simulink model "fw_pos_control"  (R2024b)
settings: Solver=VariableStepAuto  StartTime=0.0  StopTime=10.0  RelTol=1e-3
undefined symbols (not defined in the file): FW_AIRSPD_MIN, FW_ARSP_MODE, FW_L1_DAMPING, FW_L1_PERIOD, FW_L1_R_SLEW_MAX, FW_POSCTL_INV_ST, FW_R_LIM, RWTO_AIRSPD_SCL, RWTO_RAMP_TIME
libraries: simulink_extras x10, matrix_library x7, simulink x3
settings Model: DataDictionary=nextpilot_datadict.sldd  Creator=CETCA  LastModifiedBy=cetca

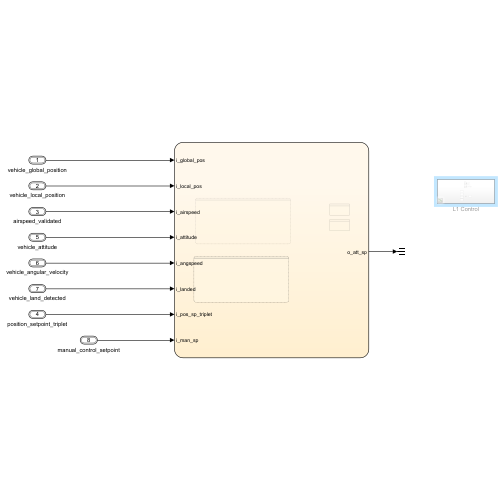
[thumbnail: Simulink's stored preview of the top-level diagram]
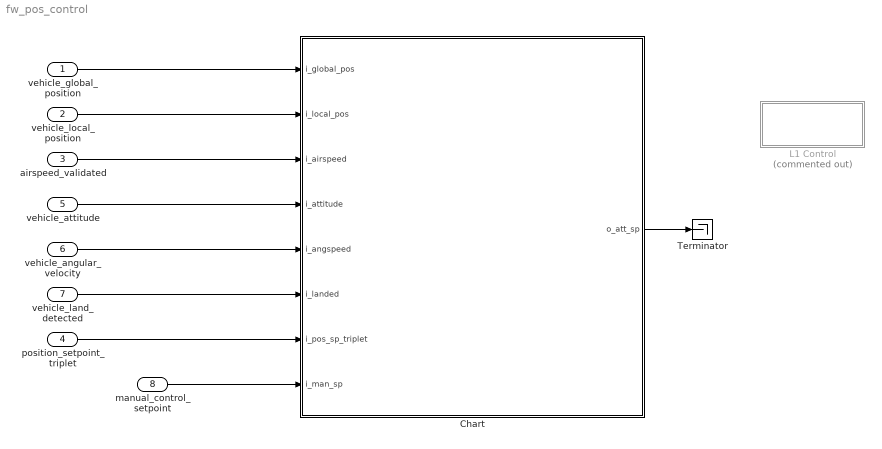
== system fw_pos_control ==
  vehicle_global_position : Inport  OutDataTypeStr=Bus: vehicle_global_position_s
  vehicle_local_position : Inport  Port=2  OutDataTypeStr=Bus: vehicle_local_position_s
  airspeed_validated : Inport  Port=3  OutDataTypeStr=Bus: airspeed_validated_s
  position_setpoint_triplet : Inport  Port=4  OutDataTypeStr=Bus: position_setpoint_triplet_s
  vehicle_attitude : Inport  Port=5  OutDataTypeStr=Bus: vehicle_attitude_s
  vehicle_angular_velocity : Inport  Port=6  OutDataTypeStr=Bus: vehicle_angular_velocity_s
  vehicle_land_detected : Inport  Port=7  OutDataTypeStr=Bus: vehicle_land_detected_s
  manual_control_setpoint : Inport  Port=8  OutDataTypeStr=Bus: manual_control_setpoint_s
  Chart : Stateflow chart  TreatAsAtomicUnit=on
  L1 Control : Subsystem  Commented=on
  Terminator : Terminator
  wires:
  vehicle_attitude/1 -> Chart/4(i_attitude)
  vehicle_angular_velocity/1 -> Chart/5(i_angspeed)
  vehicle_land_detected/1 -> Chart/6(i_landed)
  vehicle_global_position/1 -> Chart/1(i_global_pos)
  vehicle_local_position/1 -> Chart/2(i_local_pos)
  airspeed_validated/1 -> Chart/3(i_airspeed)
  position_setpoint_triplet/1 -> Chart/7(i_pos_sp_triplet)
  Chart/1(o_att_sp) -> Terminator/1
  manual_control_setpoint/1 -> Chart/8(i_man_sp)

== system fw_pos_control/Chart/L1.navigate_heading ==
  f : TriggerPort  TriggerType=function-call  VariantControl=(inherit)
      settings: CopyFcn=Stateflow.SLINSF.SimulinkMan.removeBlockPreDeleteFcn  PreDeleteFcn=Stateflow.SLINSF.SimulinkMan.unsafePredeleteFcn
  Ground : Ground
  nav_bearing : Outport
  bearing_error : Outport  Port=2
  target_bearing : Outport  Port=3
  wires:
  Ground/1 -> target_bearing/1, bearing_error/1, nav_bearing/1

== system fw_pos_control/Chart/L1.navigate_waypoints ==
  f : TriggerPort  TriggerType=function-call  VariantControl=(inherit)
      settings: CopyFcn=Stateflow.SLINSF.SimulinkMan.removeBlockPreDeleteFcn  PreDeleteFcn=Stateflow.SLINSF.SimulinkMan.unsafePredeleteFcn

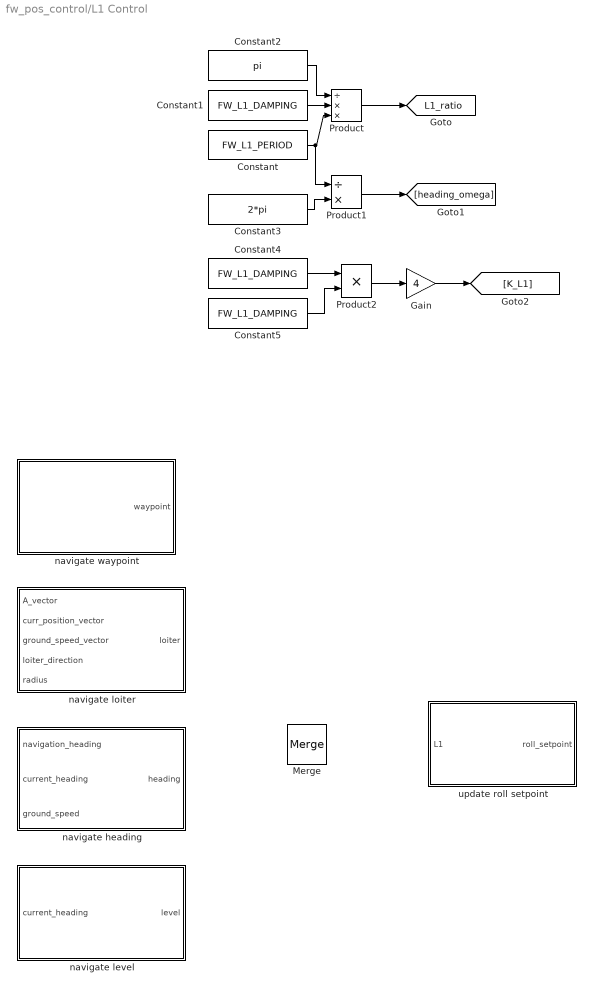
== system fw_pos_control/L1 Control ==
  Constant : Constant  Value=FW_L1_PERIOD
  Constant1 : Constant  Value=FW_L1_DAMPING
  Constant2 : Constant  Value=pi
  Constant3 : Constant  Value=2*pi
  Constant4 : Constant  Value=FW_L1_DAMPING
  Constant5 : Constant  Value=FW_L1_DAMPING
  Gain : Gain  Gain=4
  Merge : Merge  Inputs=4
  Product : Product  Inputs=/**
  Product1 : Product  Inputs=/*
  Product2 : Product
  navigate heading : Subsystem
  navigate level : Subsystem
  navigate loiter : Subsystem
  navigate waypoint : Subsystem
  update roll setpoint : Subsystem
  tag scope: L1_ratio=global
  wires:
  Constant2/1 -> Product/1
  Product/1 -> [L1_ratio]
  Constant1/1 -> Product/2
  Constant/1 -> Product1/1, Product/3
  Constant3/1 -> Product1/2
  Product1/1 -> [heading_omega]
  Constant4/1 -> Product2/1
  Constant5/1 -> Product2/2
  Product2/1 -> Gain/1
  Gain/1 -> [K_L1]

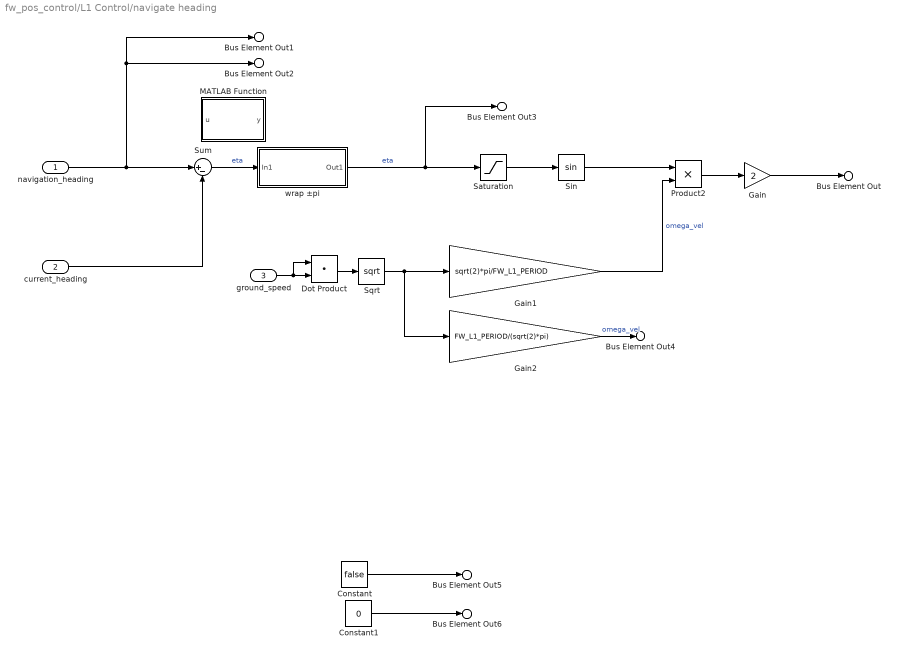
== system fw_pos_control/L1 Control/navigate heading ==
  navigation_heading : Inport
  current_heading : Inport  Port=2
  ground_speed : Inport  Port=3
  Constant : Constant  Value=false
  Constant1 : Constant  Value=0
  Dot Product : DotProduct  OutDataTypeStr=Inherit: Inherit via internal rule
  Gain : Gain  Gain=2
  Gain1 : Gain  Gain=sqrt(2)*pi/FW_L1_PERIOD
  Gain2 : Gain  Gain=FW_L1_PERIOD/(sqrt(2)*pi)
  MATLAB Function : MATLAB Function  TreatAsAtomicUnit=on
  Product2 : Product
  Saturation : Saturate  UpperLimit=pi/2  LowerLimit=-pi/2
      settings: AttributesFormatString=[%<LowerLimit>,%<UpperLimit>]
  Sin : Trigonometry
  Sqrt : Sqrt
  Sum : Sum  Inputs=|+-
  wrap ±pi : Subsystem
  Bus Element Out : Outport  PortName=heading  Element=lateral_accel
  Bus Element Out1 : Outport  PortName=heading  Element=target_bearing
  Bus Element Out2 : Outport  PortName=heading  Element=nav_bearing
  Bus Element Out3 : Outport  PortName=heading  Element=bearing_error
  Bus Element Out4 : Outport  PortName=heading  Element=L1_distance
  Bus Element Out5 : Outport  PortName=heading  Element=circle_mode
  Bus Element Out6 : Outport  PortName=heading  Element=crosstrack_error
  wires:
  navigation_heading/1 -> Bus Element Out2/1, Bus Element Out1/1, Sum/1
  current_heading/1 -> Sum/2
  wrap ±pi/1(Out1) -> Bus Element Out3/1, Saturation/1  "eta"
  Saturation/1 -> Sin/1
  ground_speed/1 -> Dot Product/2, Dot Product/1
  Sqrt/1 -> Gain2/1, Gain1/1
  Constant/1 -> Bus Element Out5/1
  Constant1/1 -> Bus Element Out6/1
  Sin/1 -> Product2/1
  Product2/1 -> Gain/1
  Sum/1 -> wrap ±pi/1(In1)  "eta"
  Dot Product/1 -> Sqrt/1
  Gain1/1 -> Product2/2  "omega_vel"
  Gain2/1 -> Bus Element Out4/1  "omega_vel"
  Gain/1 -> Bus Element Out/1

== system fw_pos_control/L1 Control/navigate level ==
  current_heading : Inport
  Constant : Constant  Value=false
  Constant1 : Constant  Value=0
  Bus Element Out : Outport  PortName=level  Element=target_bearing
  Bus Element Out1 : Outport  PortName=level  Element=nav_bearing
  Bus Element Out2 : Outport  PortName=level  Element=bearing_error
  Bus Element Out3 : Outport  PortName=level  Element=crosstrack_error
  Bus Element Out4 : Outport  PortName=level  Element=lateral_accel
  Bus Element Out5 : Outport  PortName=level  Element=circle_mode
  wires:
  Constant/1 -> Bus Element Out5/1
  Constant1/1 -> Bus Element Out3/1, Bus Element Out4/1, Bus Element Out2/1
  current_heading/1 -> Bus Element Out1/1, Bus Element Out/1

== system fw_pos_control/L1 Control/navigate loiter ==
  A_vector : Inport
  curr_position_vector : Inport  Port=2
  ground_speed_vector : Inport  Port=3
  loiter_direction : Inport  Port=4
  radius : Inport  Port=5
  Capture Mode : Subsystem
  Subsystem : Subsystem
  Bus Element Out : Outport  PortName=loiter  Element=signal1
  wires:
  ground_speed_vector/1 -> Subsystem/1(ground_speed_vector)
  Subsystem/1(guidance) -> Capture Mode/1(guidance)
  radius/1 -> Capture Mode/3(radius)
  loiter_direction/1 -> Capture Mode/2(loiter_direction)
  curr_position_vector/1 -> Subsystem/2(curr_position_vector)
  A_vector/1 -> Subsystem/3(coc_vector)

== system fw_pos_control/L1 Control/navigate waypoint ==
  Subsystem : Subsystem
  Subsystem1 : Subsystem
  Bus Element Out : Outport  PortName=waypoint  Element=signal1
  wires:
  Subsystem1/1(guidance) -> Subsystem/1(guidance)

== system fw_pos_control/L1 Control/update roll setpoint ==
  Bus Element In : Inport  PortName=L1  Element=lateral_accel
  Atan : Trigonometry  Operator=atan
  Gain : Gain  Gain=1/9.81
  Rate Limiter : RateLimiter  RisingSlewLimit=FW_L1_R_SLEW_MAX  FallingSlewLimit=-FW_L1_R_SLEW_MAX  SampleTimeMode=inherited
      settings: AttributesFormatString=[%<FallingSlewLimit>,%<RisingSlewLimit>]
  Saturation : Saturate  UpperLimit=FW_R_LIM  LowerLimit=-FW_R_LIM
      settings: AttributesFormatString=[%<LowerLimit>,%<UpperLimit>]
  roll_setpoint : Outport
  wires:
  Bus Element In/1 -> Gain/1
  Gain/1 -> Atan/1
  Atan/1 -> Saturation/1
  Saturation/1 -> Rate Limiter/1
  Rate Limiter/1 -> roll_setpoint/1

== system fw_pos_control/L1 Control/navigate heading/wrap ±pi ==
  In1 : Inport
  Bias : Bias  Bias=pi  SaturateOnIntegerOverflow=off
  Bias1 : Bias  Bias=-pi  SaturateOnIntegerOverflow=off
  Constant : Constant  Value=2*pi
  Mod : Math  Operator=mod
  Out1 : Outport
  wires:
  In1/1 -> Bias/1
  Bias/1 -> Mod/1
  Constant/1 -> Mod/2
  Mod/1 -> Bias1/1
  Bias1/1 -> Out1/1

== system fw_pos_control/L1 Control/navigate loiter/Capture Mode ==
  Bus Element In : Inport  PortName=guidance
  Bus Element In1 : Inport  PortName=guidance
  loiter_direction : Inport  Port=2
  radius : Inport  Port=3
  Check Switch Over : Subsystem
  Switch : Switch  Criteria=u2 > Threshold  SaturateOnIntegerOverflow=off  InputSameDT=off
  capture (towards waypoint center) : Subsystem
  circle (loiter) : Subsystem
  loiter_direction1 : InportShadow  Port=2
  Out1 : Outport
  wires:
  Check Switch Over/1(checkover) -> Switch/2
  capture (towards waypoint center)/1(capture) -> Check Switch Over/1(capture), Switch/1
  circle (loiter)/1(loiter) -> Check Switch Over/3(loiter), Switch/3
  Bus Element In/1 -> capture (towards waypoint center)/1(guidance)
  Bus Element In1/1 -> circle (loiter)/1(guidance)
  loiter_direction/1 -> Check Switch Over/2(direction)
  loiter_direction1/1 -> circle (loiter)/3(loiter_direction)
  radius/1 -> circle (loiter)/2(radius)
  Switch/1 -> Out1/1

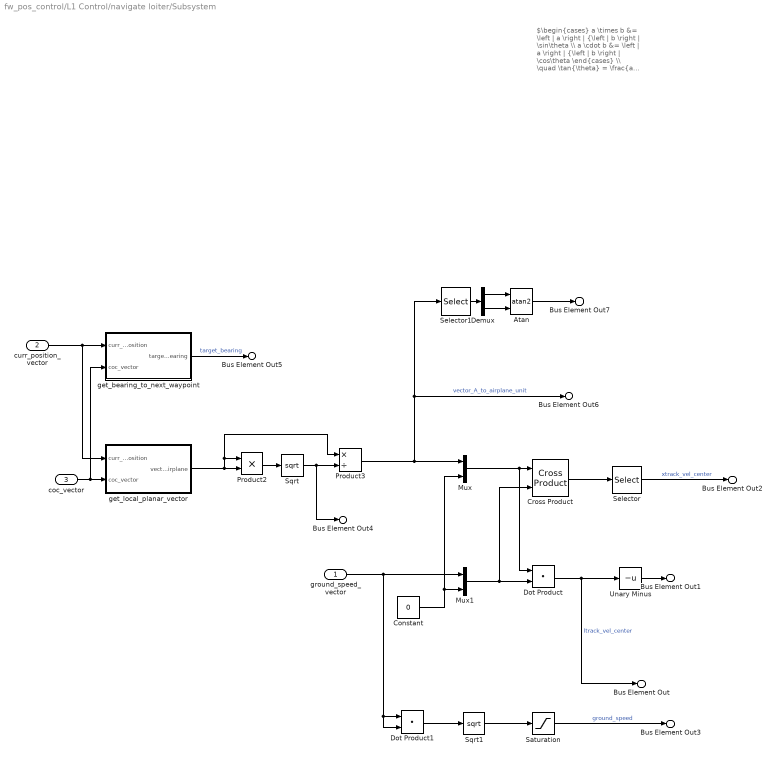
== system fw_pos_control/L1 Control/navigate loiter/Subsystem ==
  note: $\begin{cases} a \times b &= \left | a \right | {\left | b \right | \sin\theta \\ a \cdot b &= \left | a \right | {\left | b \right | \cos\theta \end{cases} \\ \quad \tan{\theta} = \frac{a \times b}{a \cdot b}$
  ground_speed_vector : Inport
  curr_position_vector : Inport  Port=2
  coc_vector : Inport  Port=3
  Atan : Trigonometry  Operator=atan2
  Constant : Constant  Value=0  OutDataTypeStr=single
  Cross Product : matrix_library/Cross Product
  Demux : Demux  Outputs=2
  Dot Product : DotProduct  OutDataTypeStr=Inherit: Inherit via internal rule
  Dot Product1 : DotProduct  OutDataTypeStr=Inherit: Inherit via internal rule
  Mux : Mux  Inputs=2
  Mux1 : Mux  Inputs=2
  Product2 : Product
  Product3 : Product  Inputs=*/
  Saturation : Saturate  UpperLimit=inf  LowerLimit=0.1
  Selector : Selector  InputPortWidth=3  IndexOptions=Index vector (dialog)  Indices=3  OutputSizes=1
  Selector1 : Selector  InputPortWidth=2  IndexOptions=Index vector (dialog)  Indices=[2 1]  OutputSizes=1
  Sqrt : Sqrt
  Sqrt1 : Sqrt
  Unary Minus : UnaryMinus
  get_bearing_to_next_waypoint : Subsystem
  get_local_planar_vector : Subsystem
  Bus Element Out : Outport  PortName=guidance  Element=xtrack_vel_circle
  Bus Element Out1 : Outport  PortName=guidance  Element=ltrack_vel_center
  Bus Element Out2 : Outport  PortName=guidance  Element=xtrack_vel_center
  Bus Element Out3 : Outport  PortName=guidance  Element=ground_speed
  Bus Element Out4 : Outport  PortName=guidance  Element=vector_A_to_airplane_length
  Bus Element Out5 : Outport  PortName=guidance  Element=target_bearing
  Bus Element Out6 : Outport  PortName=guidance  Element=vector_A_to_airplane_unit
  Bus Element Out7 : Outport  PortName=guidance  Element=nav_bearing
  wires:
  Dot Product/1 -> Bus Element Out/1, Unary Minus/1  "ltrack_vel_center"
  Unary Minus/1 -> Bus Element Out1/1
  Selector/1 -> Bus Element Out2/1  "xtrack_vel_center"
  Product3/1 -> Selector1/1, Bus Element Out6/1, Mux/1  "vector_A_to_airplane_unit"
  ground_speed_vector/1 -> Dot Product1/2, Dot Product1/1, Mux1/1
  Constant/1 -> Mux/2, Mux1/2
  Mux/1 -> Dot Product/1, Cross Product/1
  Mux1/1 -> Cross Product/2, Dot Product/2
  Cross Product/1 -> Selector/1
  get_local_planar_vector/1(vector_A_to_airplane) -> Product3/1, Product2/1, Product2/2
  Sqrt/1 -> Bus Element Out4/1, Product3/2
  Product2/1 -> Sqrt/1
  Dot Product1/1 -> Sqrt1/1
  Sqrt1/1 -> Saturation/1
  Saturation/1 -> Bus Element Out3/1  "ground_speed"
  get_bearing_to_next_waypoint/1(target_bearing) -> Bus Element Out5/1  "target_bearing"
  curr_position_vector/1 -> get_local_planar_vector/1(curr_position), get_bearing_to_next_waypoint/1(curr_position)
  coc_vector/1 -> get_bearing_to_next_waypoint/2(coc_vector), get_local_planar_vector/2(coc_vector)
  Selector1/1 -> Demux/1
  Demux/1 -> Atan/1
  Demux/2 -> Atan/2
  Atan/1 -> Bus Element Out7/1

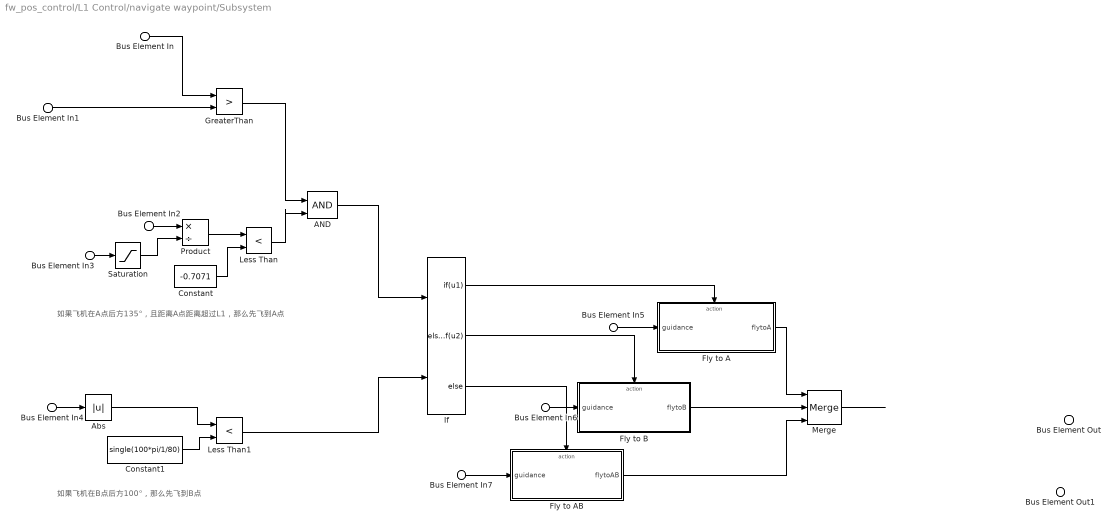
== system fw_pos_control/L1 Control/navigate waypoint/Subsystem ==
  note: 如果飞机在A点后方135°，且距离A点距离超过L1，那么先飞到A点
  note: 如果飞机在B点后方100°，那么先飞到B点
  Bus Element In5 : Inport  PortName=guidance
  Bus Element In6 : Inport  PortName=guidance
  Bus Element In7 : Inport  PortName=guidance
  Bus Element In : Inport  PortName=guidance  Element=distance_A_to_airplane
  Bus Element In3 : Inport  PortName=guidance  Element=distance_A_to_airplane
  Bus Element In2 : Inport  PortName=guidance  Element=alongTrackDist
  Bus Element In4 : Inport  PortName=guidance  Element=AB_to_BP_bearing
  Bus Element In1 : Inport  PortName=guidance  Element=L1_distance
  AND : Logic  IconShape=distinctive  AllPortsSameDT=off  OutDataTypeStr=boolean
  Abs : Abs  SaturateOnIntegerOverflow=off
  Constant : Constant  Value=-0.7071  OutDataTypeStr=single
  Constant1 : Constant  Value=single(100*pi/1/80)  OutDataTypeStr=single
  Fly to A : Subsystem  TreatAsAtomicUnit=on
  Fly to AB : Subsystem  TreatAsAtomicUnit=on
  Fly to B : Subsystem  TreatAsAtomicUnit=on
  GreaterThan : RelationalOperator  Operator=>  OutDataTypeStr=boolean  RndMeth=Simplest  InputSameDT=off
  If : If  NumInputs=2  IfExpression=u1  ElseIfExpressions=u2
  Less Than : RelationalOperator  Operator=<  OutDataTypeStr=boolean  RndMeth=Simplest  InputSameDT=off
  Less Than1 : RelationalOperator  Operator=<  OutDataTypeStr=boolean  RndMeth=Simplest  InputSameDT=off
  Merge : Merge  Inputs=3
  Product : Product  Inputs=*/
  Saturation : Saturate  UpperLimit=inf  LowerLimit=1
  Bus Element Out : Outport  PortName=OutBus  Element=bearing_error
  Bus Element Out1 : Outport  PortName=OutBus  Element=bearing_error1
  wires:
  Bus Element In/1 -> GreaterThan/1
  Bus Element In2/1 -> Product/1
  Bus Element In3/1 -> Saturation/1
  Saturation/1 -> Product/2
  Product/1 -> Less Than/1
  Constant/1 -> Less Than/2
  GreaterThan/1 -> AND/1
  Less Than/1 -> AND/2
  Bus Element In4/1 -> Abs/1
  Constant1/1 -> Less Than1/2
  Less Than1/1 -> If/2
  AND/1 -> If/1
  If/1 -> Fly to A/Action
  If/2 -> Fly to B/Action
  If/3 -> Fly to AB/Action
  Abs/1 -> Less Than1/1
  Bus Element In5/1 -> Fly to A/1(guidance)
  Bus Element In6/1 -> Fly to B/1(guidance)
  Bus Element In7/1 -> Fly to AB/1(guidance)
  Fly to A/1(flytoA) -> Merge/1
  Fly to B/1(flytoB) -> Merge/2
  Fly to AB/1(flytoAB) -> Merge/3
  Bus Element In1/1 -> GreaterThan/2
  Merge/1 -> ?

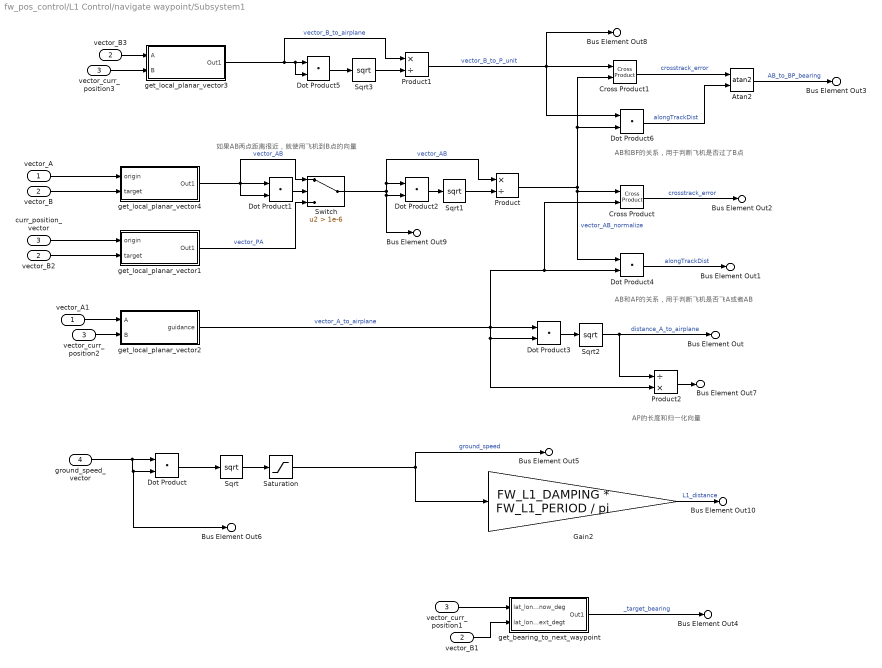
== system fw_pos_control/L1 Control/navigate waypoint/Subsystem1 ==
  note: AP的长度和归一化向量
  note: AB和AP的关系，用于判断飞机是否飞A或者AB
  note: AB和BP的关系，用于判断飞机是否过了B点
  note: 如果AB两点距离很近，就使用飞机到B点的向量
  vector_A : Inport
  vector_B : Inport  Port=2
  curr_position_vector : Inport  Port=3
  ground_speed_vector : Inport  Port=4
  Atan2 : Trigonometry  Operator=atan2
  Cross Product : matrix_library/Cross Product
  Cross Product1 : matrix_library/Cross Product
  Dot Product{,1..6} (7 alike) : DotProduct  OutDataTypeStr=Inherit: Inherit via internal rule
  Gain2 : Gain  Gain=FW_L1_DAMPING * FW_L1_PERIOD / pi
  Product : Product  Inputs=*/
  Product1 : Product  Inputs=*/
  Product2 : Product  Inputs=/*
  Saturation : Saturate  UpperLimit=inf  LowerLimit=0.1
  Sqrt{,1..3} (4 alike) : Sqrt
  Switch : Switch  Criteria=u2 > Threshold  Threshold=1e-6  SaturateOnIntegerOverflow=off  InputSameDT=off
  get_bearing_to_next_waypoint : Subsystem
  get_local_planar_vector1 : Subsystem
  get_local_planar_vector2 : Subsystem
  get_local_planar_vector3 : Subsystem
  get_local_planar_vector4 : Subsystem
  vector_A1 : InportShadow
  vector_B1 : InportShadow  Port=2
  vector_B2 : InportShadow  Port=2
  vector_B3 : InportShadow  Port=2
  vector_curr_position1 : InportShadow  Port=3
  vector_curr_position2 : InportShadow  Port=3
  vector_curr_position3 : InportShadow  Port=3
  Bus Element Out : Outport  PortName=guidance  Element=distance_A_to_airplane
  Bus Element Out1 : Outport  PortName=guidance  Element=alongTrackDist
  Bus Element Out2 : Outport  PortName=guidance  Element=crosstrack_error
  Bus Element Out3 : Outport  PortName=guidance  Element=AB_to_BP_bearing
  Bus Element Out5 : Outport  PortName=guidance  Element=ground_speed
  Bus Element Out6 : Outport  PortName=guidance  Element=ground_speed_vector
  Bus Element Out7 : Outport  PortName=guidance  Element=vector_A_to_airplane_unit
  Bus Element Out8 : Outport  PortName=guidance  Element=vector_B_to_P_unit
  Bus Element Out9 : Outport  PortName=guidance  Element=vector_AB
  Bus Element Out4 : Outport  PortName=guidance  Element=target_bearing
  Bus Element Out10 : Outport  PortName=guidance  Element=L1_distance
  wires:
  ground_speed_vector/1 -> Bus Element Out6/1, Dot Product/2, Dot Product/1
  Dot Product/1 -> Sqrt/1
  Sqrt/1 -> Saturation/1
  Saturation/1 -> Gain2/1, Bus Element Out5/1  "ground_speed"
  vector_B/1 -> get_local_planar_vector4/2(target)
  get_local_planar_vector4/1(Out1) -> Dot Product1/2, Switch/1, Dot Product1/1  "vector_AB"
  vector_curr_position1/1 -> get_bearing_to_next_waypoint/1(lat_lon_now_deg)
  vector_B1/1 -> get_bearing_to_next_waypoint/2(lat_lon_next_degt)
  get_bearing_to_next_waypoint/1(Out1) -> Bus Element Out4/1  "_target_bearing"
  vector_A/1 -> get_local_planar_vector4/1(origin)
  curr_position_vector/1 -> get_local_planar_vector1/1(origin)
  vector_B2/1 -> get_local_planar_vector1/2(target)
  get_local_planar_vector1/1(Out1) -> Switch/3  "vector_PA"
  Dot Product1/1 -> Switch/2
  Switch/1 -> Dot Product2/1, Product/1, Bus Element Out9/1, Dot Product2/2  "vector_AB"
  Dot Product2/1 -> Sqrt1/1
  Sqrt1/1 -> Product/2
  Product/1 -> Dot Product4/1, Cross Product/1, Dot Product6/2, Cross Product1/2  "vector_AB_normalize"
  vector_A1/1 -> get_local_planar_vector2/1(A)
  vector_curr_position2/1 -> get_local_planar_vector2/2(B)
  get_local_planar_vector2/1(guidance) -> Product2/2, Dot Product3/2, Cross Product/2, Dot Product4/2, Dot Product3/1  "vector_A_to_airplane"
  Cross Product/1 -> Bus Element Out2/1  "crosstrack_error"
  Dot Product3/1 -> Sqrt2/1
  Sqrt2/1 -> Product2/1, Bus Element Out/1  "distance_A_to_airplane"
  Dot Product4/1 -> Bus Element Out1/1  "alongTrackDist"
  vector_B3/1 -> get_local_planar_vector3/1(A)
  vector_curr_position3/1 -> get_local_planar_vector3/2(B)
  get_local_planar_vector3/1(Out1) -> Product1/1, Dot Product5/2, Dot Product5/1  "vector_B_to_airplane"
  Dot Product5/1 -> Sqrt3/1
  Sqrt3/1 -> Product1/2
  Product1/1 -> Bus Element Out8/1, Cross Product1/1, Dot Product6/1  "vector_B_to_P_unit"
  Cross Product1/1 -> Atan2/1  "crosstrack_error"
  Dot Product6/1 -> Atan2/2  "alongTrackDist"
  Atan2/1 -> Bus Element Out3/1  "AB_to_BP_bearing"
  Product2/1 -> Bus Element Out7/1
  Gain2/1 -> Bus Element Out10/1  "L1_distance"

== system fw_pos_control/L1 Control/navigate loiter/Capture Mode/Check Switch Over ==
  Bus Element In : Inport  PortName=capture  Element=lateral_accel
  direction : Inport  Port=2
  Bus Element In1 : Inport  Port=3  PortName=loiter  Element=lateral_accel
  Bus Element In2 : Inport  Port=3  PortName=loiter  Element=xtrack_err_circle
  AND : Logic  IconShape=distinctive  AllPortsSameDT=off  OutDataTypeStr=boolean
  Compare To Zero : simulink/Logic and Bit Operations/Compare To Zero  relop=>  OutDataTypeStr=boolean
  Compare To Zero1 : simulink/Logic and Bit Operations/Compare To Zero  relop=>  OutDataTypeStr=boolean
  Product8 : Product
  Sum : Sum  Inputs=|+-
  checkover : Outport
  wires:
  Product8/1 -> Compare To Zero/1
  Compare To Zero/1 -> AND/1
  direction/1 -> Product8/2
  Compare To Zero1/1 -> AND/2
  AND/1 -> checkover/1
  Bus Element In1/1 -> Sum/1
  Bus Element In/1 -> Sum/2
  Sum/1 -> Product8/1
  Bus Element In2/1 -> Compare To Zero1/1

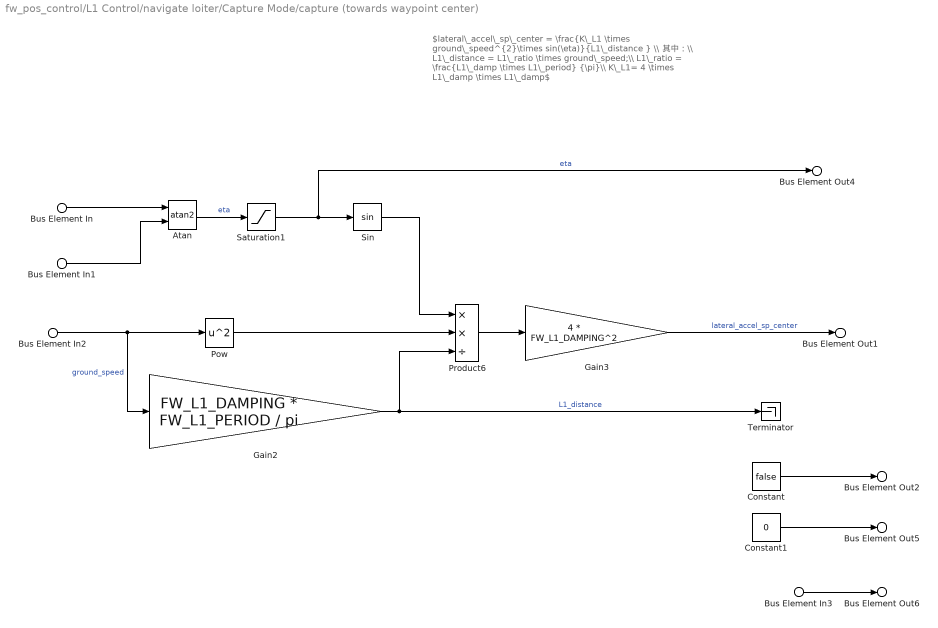
== system fw_pos_control/L1 Control/navigate loiter/Capture Mode/capture (towards waypoint center) ==
  note: $lateral\_accel\_sp\_center = \frac{K\_L1 \times ground\_speed^{2}\times sin(\eta)}{L1\_distance } \\ 其中：\\ L1\_distance = L1\_ratio \times ground\_speed;\\ L1\_ratio = \frac{L1\_damp \times L1\_period} {\pi}\\ K\_L1= 4 \times L1\_damp \times L1\_damp$
  Bus Element In : Inport  PortName=guidance  Element=xtrack_vel_center
  Bus Element In1 : Inport  PortName=guidance  Element=ltrack_vel_center
  Bus Element In2 : Inport  PortName=guidance  Element=ground_speed
  Bus Element In3 : Inport  PortName=guidance  Element=nav_bearing
  Atan : Trigonometry  Operator=atan2
  Constant : Constant  Value=false
  Constant1 : Constant  Value=0
  Gain2 : Gain  Gain=FW_L1_DAMPING * FW_L1_PERIOD / pi
  Gain3 : Gain  Gain=4 * FW_L1_DAMPING^2
  Pow : Math  Operator=square  SignedPower=on  RndMeth=Zero
  Product6 : Product  Inputs=**/
  Saturation1 : Saturate  UpperLimit=single(pi/2)  LowerLimit=-single(pi/2)
      settings: AttributesFormatString=[%<LowerLimit>,%<UpperLimit>]
  Sin : Trigonometry
  Terminator : Terminator
  Bus Element Out2 : Outport  PortName=capture  Element=circle_mode
  Bus Element Out1 : Outport  PortName=capture  Element=lateral_accel
  Bus Element Out4 : Outport  PortName=capture  Element=bearing_error
  Bus Element Out6 : Outport  PortName=capture  Element=nav_bearing
  Bus Element Out5 : Outport  PortName=capture  Element=xtrack_err_circle
  wires:
  Sin/1 -> Product6/1
  Saturation1/1 -> Bus Element Out4/1, Sin/1  "eta"
  Bus Element In2/1 -> Pow/1, Gain2/1  "ground_speed"
  Gain2/1 -> Terminator/1, Product6/3  "L1_distance"
  Gain3/1 -> Bus Element Out1/1  "lateral_accel_sp_center"
  Bus Element In1/1 -> Atan/2
  Pow/1 -> Product6/2
  Atan/1 -> Saturation1/1  "eta"
  Product6/1 -> Gain3/1
  Bus Element In/1 -> Atan/1
  Constant/1 -> Bus Element Out2/1
  Constant1/1 -> Bus Element Out5/1
  Bus Element In3/1 -> Bus Element Out6/1

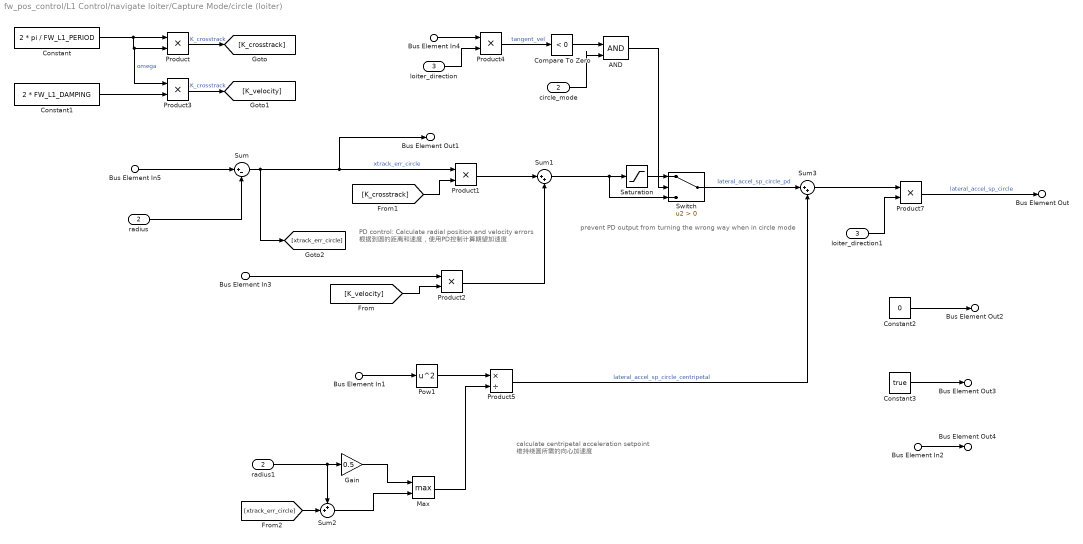
== system fw_pos_control/L1 Control/navigate loiter/Capture Mode/circle (loiter) ==
  note: prevent PD output from turning the wrong way when in circle mode
  note: calculate centripetal acceleration setpoint
      | 维持绕圆所需的向心加速度
  note: PD control: Calculate radial position and velocity errors
      | 根据到圆的距离和速度，使用PD控制计算期望加速度
  Bus Element In4 : Inport  PortName=guidance  Element=xtrack_vel_center
  Bus Element In1 : Inport  PortName=guidance  Element=xtrack_vel_center
  Bus Element In5 : Inport  PortName=guidance  Element=vector_A_to_airplane_length
  Bus Element In3 : Inport  PortName=guidance  Element=xtrack_vel_circle
  Bus Element In2 : Inport  PortName=guidance  Element=nav_bearing
  radius : Inport  Port=2
  loiter_direction : Inport  Port=3
  AND : Logic  IconShape=distinctive  AllPortsSameDT=off  OutDataTypeStr=boolean
  Compare To Zero : simulink/Logic and Bit Operations/Compare To Zero  relop=<  OutDataTypeStr=boolean
  Constant : Constant  Value=2 * pi / FW_L1_PERIOD
  Constant1 : Constant  Value=2 * FW_L1_DAMPING
  Constant2 : Constant  Value=0
  Constant3 : Constant  Value=true
  Gain : Gain  Gain=0.5
  Max : MinMax  Function=max  Inputs=2
  Pow1 : Math  Operator=square  SignedPower=on  RndMeth=Zero
  Product{,1..4,7} (6 alike) : Product
  Product5 : Product  Inputs=*/
  Saturation : Saturate  UpperLimit=inf  LowerLimit=0
  Sum : Sum  Inputs=|+-
  Sum1 : Sum  Inputs=|++
  Sum2 : Sum  Inputs=++|
  Sum3 : Sum  Inputs=|++
  Switch : Switch  Criteria=u2 > Threshold  SaturateOnIntegerOverflow=off  InputSameDT=off
  circle_mode : InportShadow  Port=2
  loiter_direction1 : InportShadow  Port=3
  radius1 : InportShadow  Port=2
  Bus Element Out3 : Outport  PortName=loiter  Element=circle_mode
  Bus Element Out : Outport  PortName=loiter  Element=lateral_accel
  Bus Element Out2 : Outport  PortName=loiter  Element=bearing_error
  Bus Element Out4 : Outport  PortName=loiter  Element=nav_bearing
  Bus Element Out1 : Outport  PortName=loiter  Element=xtrack_err_circle
  wires:
  Max/1 -> Product5/2
  Product7/1 -> Bus Element Out/1  "lateral_accel_sp_circle"
  Product4/1 -> Compare To Zero/1  "tangent_vel"
  Bus Element In3/1 -> Product2/1
  Product/1 -> [K_crosstrack]  "K_crosstrack"
  Constant/1 -> Product3/1, Product/2, Product/1  "omega"
  Product5/1 -> Sum3/2  "lateral_accel_sp_circle_centripetal"
  Pow1/1 -> Product5/1
  Sum2/1 -> Max/2
  Bus Element In4/1 -> Product4/1
  Bus Element In5/1 -> Sum/1
  Sum3/1 -> Product7/1
  Sum1/1 -> Switch/3, Saturation/1
  Sum/1 -> [xtrack_err_circle], Bus Element Out1/1, Product1/1  "xtrack_err_circle"
  loiter_direction/1 -> Product4/2
  [K_crosstrack] -> Product1/2
  loiter_direction1/1 -> Product7/2
  [K_velocity] -> Product2/2
  radius1/1 -> Gain/1, Sum2/1
  radius/1 -> Sum/2
  Product2/1 -> Sum1/2
  Gain/1 -> Max/1
  Product1/1 -> Sum1/1
  Constant1/1 -> Product3/2
  [xtrack_err_circle] -> Sum2/2
  Product3/1 -> [K_velocity]  "K_crosstrack"
  Constant2/1 -> Bus Element Out2/1
  Constant3/1 -> Bus Element Out3/1
  circle_mode/1 -> AND/2
  Compare To Zero/1 -> AND/1
  AND/1 -> Switch/2
  Saturation/1 -> Switch/1
  Switch/1 -> Sum3/1  "lateral_accel_sp_circle_pd"
  Bus Element In1/1 -> Pow1/1
  Bus Element In2/1 -> Bus Element Out4/1

== system fw_pos_control/L1 Control/navigate loiter/Subsystem/get_bearing_to_next_waypoint ==
  curr_position : Inport
  coc_vector : Inport  Port=2
  target_bearing : Outport
  wires:
  curr_position/1 -> target_bearing/1

== system fw_pos_control/L1 Control/navigate loiter/Subsystem/get_local_planar_vector ==
  curr_position : Inport
  coc_vector : Inport  Port=2
  vector_A_to_airplane : Outport
  wires:
  curr_position/1 -> vector_A_to_airplane/1

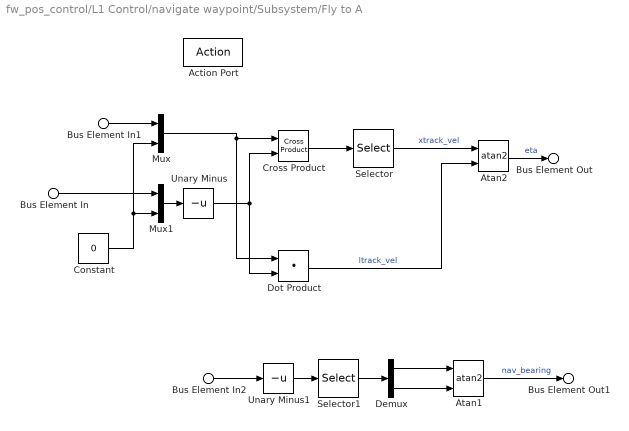
== system fw_pos_control/L1 Control/navigate waypoint/Subsystem/Fly to A ==
  Bus Element In : Inport  PortName=guidance  Element=vector_A_to_airplane_unit
  Bus Element In1 : Inport  PortName=guidance  Element=ground_speed_vector
  Bus Element In2 : Inport  PortName=guidance  Element=vector_B_to_P_unit
  Action Port : ActionPort  ActionPortLabel=if(u1)
  Atan1 : Trigonometry  Operator=atan2
  Atan2 : Trigonometry  Operator=atan2
  Constant : Constant  Value=0
  Cross Product : matrix_library/Cross Product
  Demux : Demux  Outputs=2
  Dot Product : DotProduct  OutDataTypeStr=Inherit: Inherit via internal rule
  Mux : Mux  Inputs=2
  Mux1 : Mux  Inputs=2
  Selector : Selector  InputPortWidth=3  IndexOptions=Index vector (dialog)  Indices=3  OutputSizes=1
  Selector1 : Selector  InputPortWidth=2  IndexOptions=Index vector (dialog)  Indices=[2 1]  OutputSizes=1
  Unary Minus : UnaryMinus
  Unary Minus1 : UnaryMinus
  Bus Element Out : Outport  PortName=flytoA  Element=eta
  Bus Element Out1 : Outport  PortName=flytoA  Element=nav_bearing
  wires:
  Constant/1 -> Mux/2, Mux1/2
  Bus Element In1/1 -> Mux/1
  Bus Element In/1 -> Mux1/1
  Mux/1 -> Dot Product/1, Cross Product/1
  Mux1/1 -> Unary Minus/1
  Unary Minus/1 -> Dot Product/2, Cross Product/2
  Dot Product/1 -> Atan2/2  "ltrack_vel"
  Cross Product/1 -> Selector/1
  Selector/1 -> Atan2/1  "xtrack_vel"
  Atan2/1 -> Bus Element Out/1  "eta"
  Bus Element In2/1 -> Unary Minus1/1
  Selector1/1 -> Demux/1
  Demux/2 -> Atan1/2
  Demux/1 -> Atan1/1
  Unary Minus1/1 -> Selector1/1
  Atan1/1 -> Bus Element Out1/1  "nav_bearing"

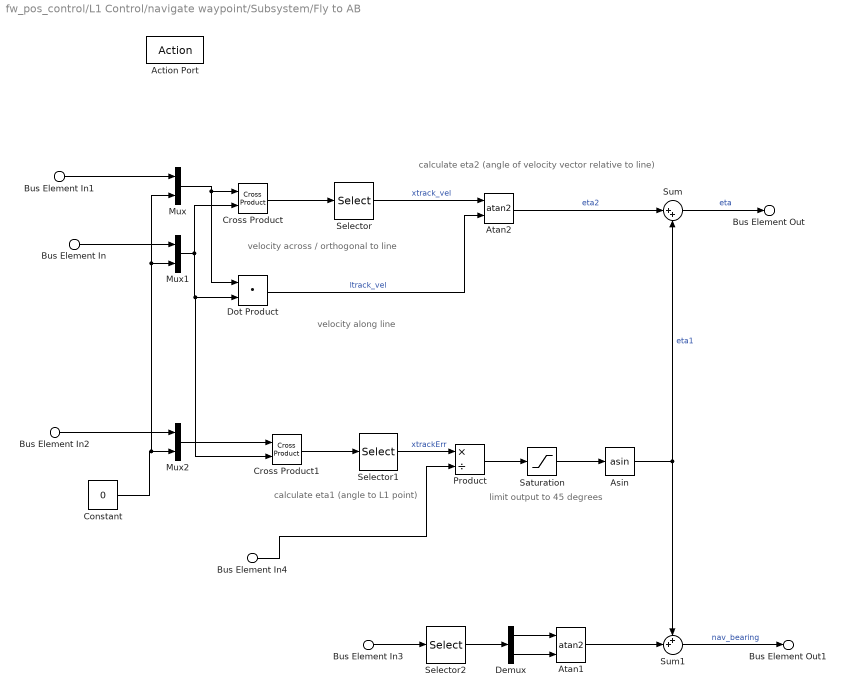
== system fw_pos_control/L1 Control/navigate waypoint/Subsystem/Fly to AB ==
  note: calculate eta1 (angle to L1 point)
  note: velocity along line
  note: velocity across / orthogonal to line
  note: calculate eta2 (angle of velocity vector relative to line)
  note: limit output to 45 degrees
  Bus Element In : Inport  PortName=guidance  Element=vector_AB
  Bus Element In3 : Inport  PortName=guidance  Element=vector_AB
  Bus Element In1 : Inport  PortName=guidance  Element=ground_speed_vector
  Bus Element In2 : Inport  PortName=guidance  Element=vector_A_to_airplane
  Bus Element In4 : Inport  PortName=guidance  Element=L1_distance
  Action Port : ActionPort  ActionPortLabel=else
  Asin : Trigonometry  Operator=asin
  Atan1 : Trigonometry  Operator=atan2
  Atan2 : Trigonometry  Operator=atan2
  Constant : Constant  Value=0
  Cross Product : matrix_library/Cross Product
  Cross Product1 : matrix_library/Cross Product
  Demux : Demux  Outputs=2
  Dot Product : DotProduct  OutDataTypeStr=Inherit: Inherit via internal rule
  Mux : Mux  Inputs=2
  Mux1 : Mux  Inputs=2
  Mux2 : Mux  Inputs=2
  Product : Product  Inputs=*/
  Saturation : Saturate  UpperLimit=sin(pi/4)  LowerLimit=-sin(pi/4)
  Selector : Selector  InputPortWidth=3  IndexOptions=Index vector (dialog)  Indices=3  OutputSizes=1
  Selector1 : Selector  InputPortWidth=3  IndexOptions=Index vector (dialog)  Indices=3  OutputSizes=1
  Selector2 : Selector  InputPortWidth=2  IndexOptions=Index vector (dialog)  Indices=[2 1]  OutputSizes=1
  Sum : Sum  Inputs=|++
  Sum1 : Sum  Inputs=++|
  Bus Element Out : Outport  PortName=flytoAB  Element=eta
  Bus Element Out1 : Outport  PortName=flytoAB  Element=nav_bearing
  wires:
  Constant/1 -> Mux/2, Mux1/2, Mux2/2
  Bus Element In1/1 -> Mux/1
  Bus Element In/1 -> Mux1/1
  Mux/1 -> Dot Product/1, Cross Product/1
  Mux1/1 -> Cross Product1/2, Dot Product/2, Cross Product/2
  Cross Product/1 -> Selector/1
  Selector/1 -> Atan2/1  "xtrack_vel"
  Dot Product/1 -> Atan2/2  "ltrack_vel"
  Atan2/1 -> Sum/1  "eta2"
  Bus Element In2/1 -> Mux2/1
  Mux2/1 -> Cross Product1/1
  Cross Product1/1 -> Selector1/1
  Selector1/1 -> Product/1  "xtrackErr"
  Product/1 -> Saturation/1
  Saturation/1 -> Asin/1
  Asin/1 -> Sum/2, Sum1/1  "eta1"
  Sum/1 -> Bus Element Out/1  "eta"
  Bus Element In3/1 -> Selector2/1
  Selector2/1 -> Demux/1
  Demux/2 -> Atan1/2
  Demux/1 -> Atan1/1
  Atan1/1 -> Sum1/2
  Sum1/1 -> Bus Element Out1/1  "nav_bearing"
  Bus Element In4/1 -> Product/2

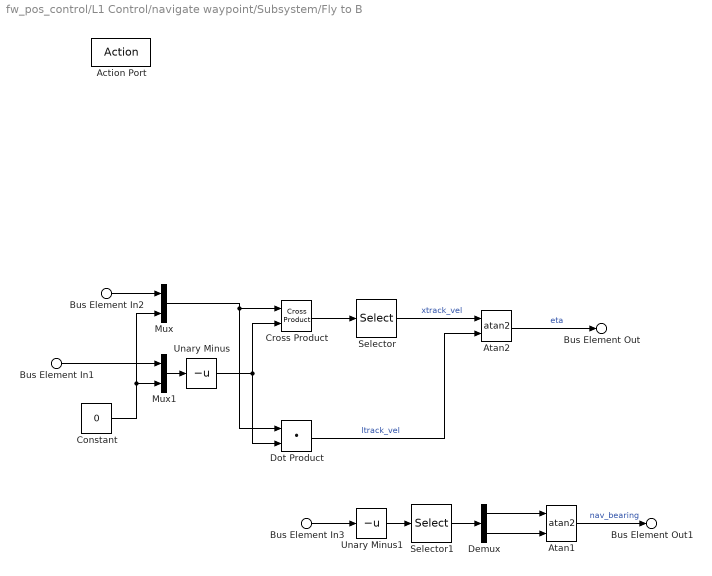
== system fw_pos_control/L1 Control/navigate waypoint/Subsystem/Fly to B ==
  Bus Element In1 : Inport  PortName=guidance  Element=vector_A_to_airplane_unit
  Bus Element In3 : Inport  PortName=guidance  Element=vector_A_to_airplane_unit
  Bus Element In2 : Inport  PortName=guidance  Element=ground_speed_vector
  Action Port : ActionPort  ActionPortLabel=elseif(..)
  Atan1 : Trigonometry  Operator=atan2
  Atan2 : Trigonometry  Operator=atan2
  Constant : Constant  Value=0
  Cross Product : matrix_library/Cross Product
  Demux : Demux  Outputs=2
  Dot Product : DotProduct  OutDataTypeStr=Inherit: Inherit via internal rule
  Mux : Mux  Inputs=2
  Mux1 : Mux  Inputs=2
  Selector : Selector  InputPortWidth=3  IndexOptions=Index vector (dialog)  Indices=3  OutputSizes=1
  Selector1 : Selector  InputPortWidth=2  IndexOptions=Index vector (dialog)  Indices=[2 1]  OutputSizes=1
  Unary Minus : UnaryMinus
  Unary Minus1 : UnaryMinus
  Bus Element Out : Outport  PortName=flytoB  Element=eta
  Bus Element Out1 : Outport  PortName=flytoB  Element=nav_bearing
  wires:
  Atan2/1 -> Bus Element Out/1  "eta"
  Dot Product/1 -> Atan2/2  "ltrack_vel"
  Mux/1 -> Dot Product/1, Cross Product/1
  Mux1/1 -> Unary Minus/1
  Selector/1 -> Atan2/1  "xtrack_vel"
  Bus Element In1/1 -> Mux1/1
  Bus Element In2/1 -> Mux/1
  Cross Product/1 -> Selector/1
  Unary Minus/1 -> Dot Product/2, Cross Product/2
  Constant/1 -> Mux/2, Mux1/2
  Demux/1 -> Atan1/1
  Atan1/1 -> Bus Element Out1/1  "nav_bearing"
  Unary Minus1/1 -> Selector1/1
  Bus Element In3/1 -> Unary Minus1/1
  Selector1/1 -> Demux/1
  Demux/2 -> Atan1/2

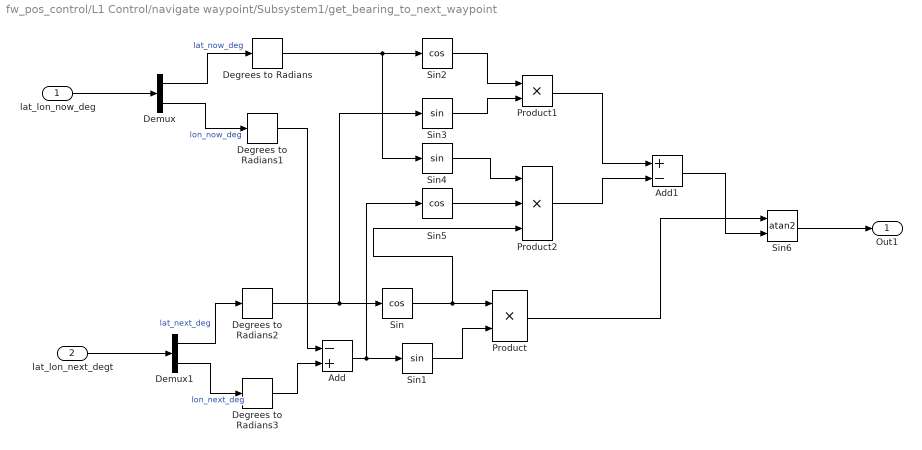
== system fw_pos_control/L1 Control/navigate waypoint/Subsystem1/get_bearing_to_next_waypoint ==
  lat_lon_now_deg : Inport
  lat_lon_next_degt : Inport  Port=2
  Add : Sum  Inputs=-+
  Add1 : Sum  Inputs=+-
  Degrees to Radians{,1..3} (4 alike) : simulink_extras/Transformations/Degrees to Radians
  Demux : Demux  Outputs=2
  Demux1 : Demux  Outputs=2
  Product : Product
  Product1 : Product
  Product2 : Product  Inputs=3
  Sin : Trigonometry  Operator=cos
  Sin1 : Trigonometry
  Sin2 : Trigonometry  Operator=cos
  Sin3 : Trigonometry
  Sin4 : Trigonometry
  Sin5 : Trigonometry  Operator=cos
  Sin6 : Trigonometry  Operator=atan2
  Out1 : Outport
  wires:
  lat_lon_now_deg/1 -> Demux/1
  lat_lon_next_degt/1 -> Demux1/1
  Demux/1 -> Degrees to Radians/1  "lat_now_deg"
  Demux/2 -> Degrees to Radians1/1  "lon_now_deg"
  Demux1/1 -> Degrees to Radians2/1  "lat_next_deg"
  Demux1/2 -> Degrees to Radians3/1  "lon_next_deg"
  Degrees to Radians2/1 -> Sin3/1, Sin/1
  Degrees to Radians1/1 -> Add/1
  Degrees to Radians3/1 -> Add/2
  Add/1 -> Sin1/1, Sin5/1
  Sin/1 -> Product2/3, Product/1
  Sin1/1 -> Product/2
  Degrees to Radians/1 -> Sin4/1, Sin2/1
  Sin2/1 -> Product1/1
  Sin3/1 -> Product1/2
  Sin4/1 -> Product2/1
  Sin5/1 -> Product2/2
  Product2/1 -> Add1/2
  Product1/1 -> Add1/1
  Sin6/1 -> Out1/1
  Product/1 -> Sin6/1
  Add1/1 -> Sin6/2

== system fw_pos_control/L1 Control/navigate waypoint/Subsystem1/get_local_planar_vector1 ==
  origin : Inport
  target : Inport  Port=2
  Add : Sum  Inputs=+-
  Add1 : Sum  Inputs=+-
  Degrees to Radians : simulink_extras/Transformations/Degrees to Radians
  Degrees to Radians1 : simulink_extras/Transformations/Degrees to Radians
  Degrees to Radians2 : simulink_extras/Transformations/Degrees to Radians
  Demux : Demux  Outputs=2
  Demux1 : Demux  Outputs=2
  Product : Product
  RADIUS_OF_EARTH1 : Gain  Gain=6371000
  RADIUS_OF_EARTH2 : Gain  Gain=6371000
  Sin2 : Trigonometry  Operator=cos
  Vector Concatenate : Concatenate
  Out1 : Outport
  wires:
  origin/1 -> Demux/1
  target/1 -> Demux1/1
  Demux/1 -> Degrees to Radians/1, Add1/2
  Add/1 -> Degrees to Radians1/1
  Add1/1 -> Degrees to Radians2/1
  Degrees to Radians/1 -> Sin2/1
  Vector Concatenate/1 -> Out1/1
  Demux1/1 -> Add1/1
  Demux1/2 -> Add/1
  Demux/2 -> Add/2
  Degrees to Radians2/1 -> RADIUS_OF_EARTH1/1  "x_angle"
  Degrees to Radians1/1 -> Product/1  "y_angle"
  Sin2/1 -> Product/2  "x_origin_cos"
  RADIUS_OF_EARTH1/1 -> Vector Concatenate/1
  Product/1 -> RADIUS_OF_EARTH2/1
  RADIUS_OF_EARTH2/1 -> Vector Concatenate/2

== system fw_pos_control/L1 Control/navigate waypoint/Subsystem1/get_local_planar_vector2 ==
  A : Inport
  B : Inport  Port=2
  guidance : Outport
  wires:
  A/1 -> guidance/1

== system fw_pos_control/L1 Control/navigate waypoint/Subsystem1/get_local_planar_vector3 ==
  A : Inport
  B : Inport  Port=2
  Out1 : Outport
  wires:
  A/1 -> Out1/1

== system fw_pos_control/L1 Control/navigate waypoint/Subsystem1/get_local_planar_vector4 ==
  origin : Inport
  target : Inport  Port=2
  Add : Sum  Inputs=+-
  Add1 : Sum  Inputs=+-
  Degrees to Radians : simulink_extras/Transformations/Degrees to Radians
  Degrees to Radians1 : simulink_extras/Transformations/Degrees to Radians
  Degrees to Radians2 : simulink_extras/Transformations/Degrees to Radians
  Demux : Demux  Outputs=2
  Demux1 : Demux  Outputs=2
  Product : Product
  RADIUS_OF_EARTH1 : Gain  Gain=6371000
  RADIUS_OF_EARTH2 : Gain  Gain=6371000
  Sin2 : Trigonometry  Operator=cos
  Vector Concatenate : Concatenate
  Out1 : Outport
  wires:
  RADIUS_OF_EARTH2/1 -> Vector Concatenate/2
  Product/1 -> RADIUS_OF_EARTH2/1
  RADIUS_OF_EARTH1/1 -> Vector Concatenate/1
  Sin2/1 -> Product/2  "x_origin_cos"
  Degrees to Radians1/1 -> Product/1  "y_angle"
  Degrees to Radians2/1 -> RADIUS_OF_EARTH1/1  "x_angle"
  Demux/2 -> Add/2
  Demux1/2 -> Add/1
  Demux1/1 -> Add1/1
  Vector Concatenate/1 -> Out1/1
  Degrees to Radians/1 -> Sin2/1
  Add1/1 -> Degrees to Radians2/1
  Add/1 -> Degrees to Radians1/1
  Demux/1 -> Add1/2, Degrees to Radians/1
  target/1 -> Demux1/1
  origin/1 -> Demux/1

== matlab function fw_pos_control/L1 Control/navigate heading/MATLAB Function ==
  data: u input; y output
function y = fcn(u)

y = u;

== stateflow chart fw_pos_control/Chart ==
  state logic_mode [parallel] [commented out]
    state init [commented out]
    state takeoff [commented out]
    init -> takeoff [commented out]
    (default) -> init [commented out]
  state L1 [group] [commented out]
    state [nav_bearing,bearing_error,target_bearing] = navigate_heading [function] [commented out]
    state navigate_waypoints [function] [commented out]
  state TECS [group] [commented out]
  state flight_mode [parallel]
    en,du:
    % 输入数据处理
    %prepare_poll_data()
    % 默认协调转弯，不使用襟翼
    o_att_sp.fw_control_yaw = false; % 航向采用协调转弯
    o_att_sp.apply_flaps       = 0; % 关闭襟翼
    settings: executionOrder=1
    note: uint8 FLAPS_OFF = 0     	# no flaps
        | uint8 FLAPS_LAND = 1    	# landing config flaps
        | uint8 FLAPS_TAKEOFF = 2 	# take-off config flaps
    state flag_control_auto [commented out]
      en,du:
      control_mode_current  = 1;
      en,du:
      state SETPOINT_TYPE_TAKEOFF [commented out]
        en:
        % 起飞时刻
        time_started_landing = getSimulationTime();
        en,du:
        % 输入变量
        curr_pos          = [0 0];
        ground_speed = [0 0];
        pos_sp_prev   = [0 0];
        pos_sp_curr    = [0 0];
        % 数据处理
        curr_wp = [pos_sp_curr.lat, pos_sp_curr.lon];
        if pos_sp_prev.valid
        prev_wp = [pos_sp_prev.lat, pos_sp_prev,lon];
        else
        prev_wp = [pos_sp_curr.lat, pos_sp_curr,lon];
        end
        % 输出变量
        att_sp.apply_flaps = uint8(2);
        state runway_takeoff_disable [commented out]
        state runway_takeoff_enable [commented out]
          en:
          % 跑道起点
          start_wp = [current_lat, current_lon];
          % 跑道海拔
          takeoff_ground_alt = current_altitude;
          % 跑道方向（根据机头航向，但是不准确）
          runway_heading = yaw;
          en,du:
          % 地形高度
          terrain_alt = takeoff_ground_alt;
          note: 爬升到安全高度
              | 1、滚转：0
              | 2、俯仰：TECS
              | 3、偏航：跑道航向
              | 4、油门：TECS
          note: 滑跑加速到离地
              | 1、滚转：0
              | 2、俯仰：RWTO_PSP
              | 3、偏航：跑道航向
              | 4、油门：RWTO_MAX_THR
          note: 离场爬升（正常固定翼飞行）
              | 1、滚转：L1控制
              | 2、俯仰：TECS
              | 3、偏航：协调转弯
              | 4、油门：TECS
          note: 油门加速
              | 1、滚转：0
              | 2、俯仰：RWTO_PSP
              | 3、偏航：跑道航向
              | 4、油门：线性增加到RWTO_MAX_THR
          state INIT [commented out]
            en:
            % 输出变量
            att_sp.roll_body = single(0.0);
            att_sp.pitch_body = RWTO_PSP;
            att_sp.yaw_body = runway_heading;
            att_sp.throttle = 0;
            att_sp.fw_control_yaw = true;
            %
            att_sp.roll_reset_integral=true;
            att_sp.pitch_reset_integral = true;
          state THROTTLE_RAMP [commented out]
            en:
            % 输出变量
            att_sp.roll_body = single(0.0);
            att_sp.pitch_body = RWTO_PSP;
            att_sp.yaw_body = runway_heading;
            att_sp.throttle = 0;
            att_sp.fw_control_yaw = true;
          state CLAMPED_TO_RUNWAY [commented out]
            en,du:
            % 输出变量
            att_sp.roll_body  = single(0.0);
            att_sp.pitch_body  = RWTO_PSP;
            att_sp.yaw_body = runway_heading;
            att_sp.throttle = min(...
            elapsed(sec)/RWTO_RAMP_TIME*RWTO_MAX_THR,...
            RWTO_MAX_THR)
            att_sp.fw_control_yaw = true;
          state TAKEOFF [commented out]
            en,du:
            % 输出变量
            att_sp.roll_body  = single(0.0);
            %att_sp.pitch_body  = TECS;
            att_sp.yaw_body = runway_heading;
            %att_sp.throttle =TECS;
            att_sp.fw_control_yaw = true;
            % 离地之后，积分器可以启用
            att_sp.roll_reset_integral=false;
            att_sp.pitch_reset_integral = false;
          state CLIMBOUT [commented out]
            en:
            if RWO_HDG == 0
            start_wp(1) = current_lat;
            start_wp(2) = current_lon;
            end
            ex:
            climbout = false;
            %
            %att_sp.roll_body = L1
            %att_sp.pitch_body=TECS
            %att_sp.yaw_body协调转弯
            %att_sp.throttle=TECS
            att_sp.fw_control_yaw = false;
          state FLY [commented out]
          (default) -> INIT [commented out]
          CLAMPED_TO_RUNWAY -> TAKEOFF [commented out] : [airspeed > FW_AIRSPD_MIN * RWTO_AIRSPD_SCL]
          INIT -> THROTTLE_RAMP [commented out]
          TAKEOFF -> CLIMBOUT [commented out] : [alt_agl > RWTO_NAV_ALT]
          THROTTLE_RAMP -> CLAMPED_TO_RUNWAY [commented out] : [after(RWTO_RAMP_TIME, sec) || ...
              | airspeed > FW_AIRSPD_MIN * RWTO_AIRSPD_SCL]
          CLIMBOUT -> FLY [commented out] : [alt_agl > FW_CLMBOUT_DIFF]
        (default) -> runway_takeoff_disable [commented out]
        runway_takeoff_disable -> runway_takeoff_enable [commented out] : [RWTO_TKOFF>0]
      state SETPOINT_TYPE_POSITION [commented out]
        en,du:
        % 计算到目标点的距离
        % 主要是计算高度
      state SETPOINT_TYPE_LOITER [commented out]
        en,du:
        % 获取盘旋半径和方向
        loiter_radius     = pos_sp_curr.loiter_radius;
        loiter_direction = pos_sp_curr.loiter_direction;
        if abs(loiter_radius) < eps
        loiter_radius = NAV_LOITER_RAD;
        loiter_direction = sign(loiter_radius);
        end
        % 调用L1库
        L1.navigate_loiter(curr_wp, curr_pos, loiter_radius, loiter_direction, nav_speed_2d);
      state SETPOINT_TYPE_LAND [commented out]
        en:
        time_started_landing = getSimulationTime();
        en,du:
        % 数据处理
        curr_wp = [pos_sp_curr.lat, pos_sp_curr.lon];
        if pos_sp_prev.valid
        prev_wp = [pos_sp_prev.lat, pos_sp_prev,lon];
        else
        prev_wp = [pos_sp_curr.lat, pos_sp_curr,lon];
        end
        % 飞机到目标点的航向
        bearing_airplane_currwp = get_bearing_to_next_waypoint(...
        curr_pos(1), curr_pos(2), curr_wp(1), curr_wp(2));
        % 上航点到目标点的航向
        if pos_sp_prev.valid
        bearing_lastwp_currwp = get_bearing_to_next_waypoint(...
        prev_wp(1), prev(2), curr_wp(1), curr_wp(2));
        else
        bearing_lastwp_currwp = bearing_airplane_currwp;
        end
        % 飞机到着陆点的距离
        wp_distance = get_distance_to_next_waypoint(...
        curr_pos(1), curr_pos(2),  curr_wp(1),  curr_wp(2))
        % 输出变量
        att_sp.apply_flaps = uint8(1);
        note: ?
        state landslope [group] [commented out]
        note: 拉漂曲线是一个指数函数
            | $f(x) = (H1+H2) exp(-\frac{tan\theta}{H1+H2}x) - H1 \\ 其中 \\ H1 = FW\_LND\_HVIRT,虚拟落地高度 \\ H2 = FW\_LND\_FLALT,拉漂高度 \\ 曲线满足\\ （1）f(0)=H2\\ （2）f'(0)=-tan(\theta)\\$
        state start_flare [commented out]
          en:
          land_noreturn_vertical=true;
        state glide_slope [commented out]
          en:
          land_noreturn_vertical=false;
        state normal_navigation [commented out]
          en:
          land_noreturn_horizontal=false;
          en,du:
          L1.navigate_waypoints()
        state heading_hold [commented out]
          en:
          land_noreturn_horizontal=true;
          en,du:
          L1.navigate_heading()
        (default) -> glide_slope [commented out]
        glide_slope -> start_flare [commented out]
        (default) -> normal_navigation [commented out]
        normal_navigation -> heading_hold [commented out] : [wp_distance<FW_LND_HHDIST
            | || ...land_noreturn_vertical]
      state SETPOINT_TYPE_IDLE [commented out]
        en,du:
        att_sp_.thrust_body(1) = single(0.0);
        att_sp_.roll_body          = single(0.0);
        att_sp_.pitch_body       = single(FW_PSP_OFF*pi/180);
      (default) -> (junction 34) [commented out]
      flag_control_auto -> (junction 34) [commented out]
      (junction 34) -> SETPOINT_TYPE_TAKEOFF [commented out]
      (junction 34) -> (junction 25) [commented out]
      SETPOINT_TYPE_TAKEOFF -> SETPOINT_TYPE_POSITION [commented out] : [~in_takeoff_situation() && airspeed >= FW_AIRSPD_MIN]
      (junction 25) -> SETPOINT_TYPE_POSITION [commented out]
      (junction 25) -> (junction 28) [commented out]
      SETPOINT_TYPE_LOITER -> SETPOINT_TYPE_POSITION [commented out]
      SETPOINT_TYPE_POSITION -> SETPOINT_TYPE_LOITER [commented out]
      (junction 28) -> SETPOINT_TYPE_LOITER [commented out]
      (junction 28) -> (junction 31) [commented out]
      (junction 31) -> SETPOINT_TYPE_LAND [commented out]
      (junction 31) -> (junction 109) [commented out]
      (junction 109) -> SETPOINT_TYPE_IDLE [commented out]
    state flag_manul_pos [commented out]
    state flag_manul_alt [commented out]
    state flag_control_idle [commented out]
    (default) -> (junction 5) [commented out]
    flight_mode -> (junction 5) [commented out]
    (junction 5) -> flag_control_auto [commented out] : [control_mode_.flag_control_auto_enabled]
    (junction 5) -> (junction 7) [commented out]
    (junction 7) -> flag_manul_pos [commented out] : [control_mode_.flag_control_velocity_enabled &&
        | control_mode_.flag_control_altitude_enabled]
    (junction 7) -> (junction 10) [commented out]
    (junction 10) -> flag_manul_alt [commented out] : [control_mode_.flag_control_altitude_enabled]
    (junction 10) -> (junction 13) [commented out]
    (junction 13) -> flag_control_idle [commented out]
  data: nav_bearing function_output double size=1; bearing_error function_output double size=1; target_bearing function_output double size=1; wp_radius function_input; dist function_output; airspeed local; alt_agl local; current_lat local; current_lon local; flag function_output; flag function_output; h function_output; h function_output; RWTO_RAMP_TIME parameter; RWTO_AIRSPD_SCL parameter; FW_AIRSPD_MIN parameter; i_global_pos input; i_local_pos input; i_airspeed input; i_attitude input; i_angspeed input; i_landed input; i_pos_sp_triplet input; o_att_sp output Bus: vehicle_attitude_setpoint_s; i_man_sp input; FW_ARSP_MODE parameter; FW_POSCTL_INV_ST parameter
  function dist = switch_distance(wp_radius):
    | function dist = switch_distance(wp_radius)
    |  
    | 
    | dist = min(wp_radius);
  function prepare_poll_data:
    | function prepare_poll_data
    | 
    | 
    | 
    | %% 空速
    | persistent airspeed_valid_time;
    | 
    | g_airspeed_valid = false;
    | g_eas_to_tas     = single(1.0);
    | 
    | if (FW_ARSP_MODE == single(0)) && ...
    |         (isfinite(i_airspeed.calibrated_airspeed_m_s) && ...
    |         (isfinite(i_airspeed.true_airspeed_m_s)) && ...
    |         (i_airspeed.calibrated_airspeed_m_s > single(0.0)))
    | 
    |     g_airspeed_valid     = true;
    |     airspeed_valid_time = uint64(getSimulationTime());
    | 
    |     airspeed_   = i_airspeed.calibrated_airspeed_m_s;
    |     g_eas_to_tas = constrain(i_airspeed.true_airspeed_m_s / i_airspeed.calibrated_airspeed_m_s, 0.9, 2.0);
    | elseif(g_airspeed_valid && (uint64(getSimulationTime()) - airspeed_valid_time > 1)) % 空速计数据持续1s无效
    |     % no airspeed updates for one second
    |     g_airspeed_valid     = false;
    |     airspeed_valid_time = uint64(0);
    | end
    | 
    | %% 手动
    | % FW_POSCTL_INV_ST, default 0
    | % @value 0 Normal stick configuration (airspeed on throttle stick, altitude on pitch stick)
    | % @value 1 Alternative stick configuration (altitude on throttle stick, airspeed on pitch stick)
    | % value 0 油门控空速，俯仰控高度，默认方式
    | % value 1 可选配置，油门控高度，俯仰控空速
    | if FW_POSCTL_INV_ST > 0.5
    |     % Alternate stick allocation (similar concept as for multirotor systems:
    |     % demanding up/down with the throttle stick, and move faster/break with the pitch one.
    |     %
    |     g_man_sp_altitude = -(constrain(i_man_sp.z, 0.0, 1.0) * 2. - 1.);
    |     g_man_sp_airspeed = constrain(i_man_sp.x, -1.0, 1.0) / 2. + 0.5;
    | else
    |     g_man_sp_altitude = i_man_sp.x;
    |     g_man_sp_airspeed = constrain(i_man_sp.z, 0.0, 1.0);
    | end
    | 
    | %% 姿态
    | % R是表示机体到大地的方向余弦
    | R = quat2dcm(i_attitude.q);
    | [g_roll, g_pitch, g_yaw] = dcm2elu(R);
    | % 体轴系的加速度和速度
    | g_body_acceleration = R' * [local_pos_.x;local_pos_.y;local_pos_.z];
    | g_body_velocity     = R' * [local_pos_.vx;local_pos_.vy;local_pos_.vz];
  function flag = in_takeoff_situation:
    | function flag = in_takeoff_situation
    | 
    | flag = (getSimulationTime() - time_went_in_air < 10) &&...
    |     (current_altitude <= takeoff_ground_alt + FW_CLMBOUT_DIFF);
  function flag = loiter_or_position:
    | function flag = loiter_or_position()
    | 
    | acc_rad = L1.switch_distance(single(500.0));
    | 
    | %获取当前位置到目标点的距离
    | [dist, dist_xy, dist_z] = get_distance_to_point_global_wgs84(...
    |     curr_wp(1), curr_wp(2), pos_sp_curr.alt,...
    |     current_latitude, current_longitude, current_altitude);
    | 
    | % FW_CLMBOUT_DIFF=10m
    | 
    | if type == 0
    |     % 水平先到了，高度还没到
    |     % 高度误差大于2倍FW_CLMBOUT_DIFF，但是水平距离小于2倍可接受的距离以内，飞机改为盘旋的方式靠近当前航点
    |     flag = (dist > 0.0) ...
    |         && (dist_z > 2.0 * FW_CLMBOUT_DIFF) ...
    |         && (dist_xy < 2.0 * max(acc_rad, abs(pos_sp_triplet.current.loiter_radius)));
    | else
    |     % 水平和高度都没到
    |      % 高度误差大于2倍FW_CLMBOUT_DIFF，且水平距离大于2倍可接受的距离以内，飞机改为航点的方式靠近当前航点
    |     flag = (dist >= 0.0) ...
    |         && (dist_z > 2.0 * FW_CLMBOUT_DIFF) ...
    |         && (dist_xy > 2.0 * max(acc_rad, abs(pos_sp_curr.loiter_radius)));
    | end
  function h = flare_relative_alt:
    | function h = flare_relative_alt
    |  h = FW_LND_FLALT;
  function h = motor_lim_relative_alt:
    | function h = motor_lim_relative_alt()
    | % check if negative value for 2/3 of flare altitude is set for throttle cut
    | % h = single(FW_LND_TLALT);    % 推力限制高度，默认-1
    | 
    | if (FW_THR_LND_MAX > 0.0)
    |     h = single(FW_THR_LND_MAX);
    | else
    |     h = single(2/3 * FW_LND_FLALT);
    | end
